simulink library "EngineSystemSubmodelVer1_0"  (R2013a)
settings: Solver=ode45  StartTime=0.0  StopTime=10.0  FixedStep=1e-4  RelTol=1e-3
values from neighbouring files (symbols this model uses):
  B = [B1;B2]    [GensetRespOptimiztion.m]    (also in GensetRespOptimiztionTorstein.m; Init8RTFLEX68D.m = 0.68; init_MVM.m = 0.127)
  beta = 0.75    [Init8RTFLEX68D.m]
  cAStartRef = 104.8    [Init8RTFLEX68D.m]
  coeffMechEff = [0.135;0.155]    [Init8RTFLEX68D.m]
  comp_eff_map = [0 0 0 0 0 0 0 0 0 0 0 0 ... (250000 elements, 500x500)]    [comp_map.mat]    (also in comp_mapABB A175-35L.mat)
  comp_flow_map = [0 0 0 0 0 0 0 0 0 0 0 0 ... (250000 elements, 500x500)]    [comp_map.mat]    (also in comp_mapABB A175-35L.mat)
  D_turb_wheel = TC.TC_map.turb.D_wheel    [init_MVM.m]
  dCALiftDown = cAVVDownRef(end) - cAVVDownRef(1)    [Init8RTFLEX68D.m]
  dCALiftTopRef = 63.5    [Init8RTFLEX68D.m]
  dCALiftUp = cAVVUpRef(end) - cAVVUpRef(1)    [Init8RTFLEX68D.m]
  Dp = 0.383    [Init8RTFLEX68D.m]
  Ds = 0.079    [Init8RTFLEX68D.m]
  Dv = 0.425    [Init8RTFLEX68D.m]
  eff_coeff = [-1.0889528323728;0.91854258409396;-0.10659748546926;                     0.21229452390244;-0.053186221596493;-0.005451194709834]    [Init8RTFLEX68D.m]
  eta_turb_max = TC.TC_map.turb.eff_max    [init_MVM.m]
  flow_coeff_turb = [-1.585326540339;-4.823836967181;1.5853156139822]    [Init8RTFLEX68D.m]    (also in init_MVM.m = TC.TC_map.turb.flow_fit_coeff)
  fs = 0.0683    [Init8RTFLEX68D.m]    (also in NOxProcessGUI.m = varargin{2}; initHybrid.m; initMV.m; init_MVM.m = 0.0682925799315)
  genset = generators(1)    [runTempCyl4S.m]
  J_tc = TC.SAE_map_comp.inertia    [init_MVM.m]
  jShaft = 0    [EngineSystemParameters.m]    (also in Init8RTFLEX68D.m = 323000)
  jTC = 2    [Init8RTFLEX68D.m]
  Kb = 1*ones(engines,1)    [initHybrid.m]    (also in initMV.m; init_MVM.m = 1; init_ele.m = 1)
  Kd = 20*ones(engines,1)    [initHybrid.m]    (also in initMV.m; init_MVM.m = 10; init_ele.m = 20)
  Ki = 20*ones(engines,1)    [initHybrid.m]    (also in initMV.m; init_MVM.m = 10; init_ele.m = 20)
  Kp = 20*ones(engines,1)    [initHybrid.m]    (also in initMV.m; init_MVM.m = 10; init_ele.m = 20)
  lambdaCrank = 0.5056    [Init8RTFLEX68D.m]
  liftMax = 0.17    [Init8RTFLEX68D.m]
  Load_amp = x(4) + xRef(i)    [GetErrGensetResp.m]    (also in runsimulation.m = 0.55; runsimulationRecovery.m = InitialLoad(jj) + LoadStep(ii))
  Load_bias = x(4)    [GetErrGensetResp.m]    (also in runsimulation.m = 0.15; runsimulationRecovery.m = InitialLoad(jj))
  Load_index = 1    [GetErrGensetResp.m]    (also in runsimulation.m; runsimulationRecovery.m)
  mqfCycMax = 9.5547e-2    (= 0.095547)    [Init8RTFLEX68D.m]
  N = x*noMol    [NOxProcessGUI.m]    (also in initHybrid.m = .1*ones(engines,1); initMV.m = .1*ones(engines,1); init_ele.m = 0.1)
  n288_rep = [0 222.054 444.108 666.162 888.216 1110.27 1332.324 1554.378 1776.432 1998.486 2220.54 2442.594 ... (500 elements, 1x500)]    [comp_map.mat]
  nPort = 28    [Init8RTFLEX68D.m]
  npr = length(pr_rep)    [Init8RTFLEX68D.m]    (also in initHybrid.m; initMV.m; init_MVM.m)
  nsp = length(n288_rep)    [Init8RTFLEX68D.m]    (also in initHybrid.m; initMV.m; init_MVM.m)
  nStroke = 2    [Init8RTFLEX68D.m]
  omegat0 = RPM_TC_initial/30*pi    [init_MVM.m]
  pr_rep = [1.01 1.0150249672 1.0200499344 1.0250749016 1.0300998688 1.035124836 1.0401498032 1.0451747704 1.0501997376 1.0552247048 1.060249672 1.0652746392 ... (500 elements, 1x500)]    [comp_map.mat]
  r = 0.035    [Init8RTFLEX68D.m]
  Start_time = 50    [GetErrGensetResp.m]    (also in runsimulation.m; runsimulationRecovery.m)
  stroke = 2.72    [Init8RTFLEX68D.m]
  T_load = 1    [GetErrGensetResp.m]    (also in runsimulation.m; runsimulationRecovery.m)
  T_ref_turb = TC.TC_map.turb.T_ref    [init_MVM.m]
  u0 = 0.2    [init_MVM.m]
  Uc_opt = TC.TC_map.turb.Uc_opt    [init_MVM.m]
  w = 0.021    [Init8RTFLEX68D.m]
  wasteGateMax = 10    [Init8RTFLEX68D.m]
  wasteGateMin = 0    [Init8RTFLEX68D.m]
  wiebePara = [0.07;0.57;3.05;11;24;56.3;1.5;1;0.7]    [Init8RTFLEX68D.m]
  X = 0.07    [Init8RTFLEX68D.m]
  Y = 0.16    [Init8RTFLEX68D.m]
undefined symbols (not defined in the file or in its folder): aCrank, cAVVDownRef, cAVVUpRef, liftDownRef, liftUpRef, omega0, Td, Ti, u_max
undefined symbols (not defined in the file): BWdmExhBypass, cAlpha, cCylHT, E0A, ECyl0, hn, KbWG, KpWG, lowerCloseSPWG, m0A, mb0A, mbCyl0, mCp, mCyl0, nCyl, phi0, phi0A, phi0rad, RPM0, RPMMax, RPMT0, TiWG, upperOpenWG, V0A, vCyl0, wasteGateRatio
libraries: EngineSystemSubmodel x49, simulink x1
(part 2 of 3)

== system EngineSystemSubmodelVer1_0/AirWaterCooler ==
  pTFu : Inport
  pTFd : Inport  Port=2
  TCW : Inport  Port=3
  Demux : Demux  Outputs=3
  Demux1 : Demux  Outputs=3
  Mux : Mux  Inputs=3
  Mux1 : Mux  Inputs=3
  S-Function : S-Function  FunctionName=AirWaterCoolerPTF  Parameters=fs,Cd,A_air_path,dm_cw,coeff_T_cw_K,Cp_cw,D_cw_pipe  SFunctionModules='GetAirDensity GetAirThermalConduct GetAirViscosity GetCompCombGas_rtwutil GetHTCoeffHTX GetIdealNozzleFlow GetThdynCombGasZach rt_nonfinite rtGetInf rtGetNaN'  EnableBusSupport=off  mask{fs=fs, Cd=Cd, A_air_path=A_air_path, dm_cw=dm_cw, coeff_T_cw_K=coeff_T_cw_K, Cp_cw=Cp_cw, D_cw_pipe=D_cw_pipe}
      mask prompts: fs "Stoichiometric fuel-air ratio"; Cd "Discharge coefficient (0.8)"; A_air_path "Effective sectional area of air path (m2)"; dm_cw "Coolant flow rate (kg/s)"; coeff_T_cw_K "Coefficient for effective heat transfer area w.r.t. coolant temperature (2x1)"; Cp_cw "Specific heat capacity of coolant"; D_cw_pipe "Pipe diameter of the cooling water pipe in the cooler (m)"
  dmEmbu : Outport
  dmEmbd : Outport  Port=2
  wires:
  S-Function/6 -> Mux1/3
  S-Function/5 -> Mux1/2
  S-Function/4 -> Mux1/1
  S-Function/3 -> Mux/3
  S-Function/2 -> Mux/2
  S-Function/1 -> Mux/1
  Demux/1 -> S-Function/1
  Demux/3 -> S-Function/3
  Demux/2 -> S-Function/2
  Demux1/3 -> S-Function/6
  Demux1/1 -> S-Function/4
  Demux1/2 -> S-Function/5
  pTFd/1 -> Demux1/1
  pTFu/1 -> Demux/1
  Mux/1 -> dmEmbu/1
  Mux1/1 -> dmEmbd/1
  TCW/1 -> S-Function/7

== system EngineSystemSubmodelVer1_0/AirWaterCoolerNV ==
  pTFu : Inport
  pTFd : Inport  Port=2
  TCW : Inport  Port=3
  Bus Creator : BusCreator  Inputs=3
  Bus Creator1 : BusCreator  Inputs=3
  Bus Selector : BusSelector  OutputSignals=p,T,F
  Bus Selector1 : BusSelector  OutputSignals=p,T,F
  S-Function : S-Function  FunctionName=AirWaterCoolerPTF  Parameters=fs,Cd,A_air_path,dm_cw,coeff_T_cw_K,Cp_cw,D_cw_pipe  SFunctionModules='GetAirDensity GetAirThermalConduct GetAirViscosity GetCompCombGas_rtwutil GetHTCoeffHTX GetIdealNozzleFlow GetThdynCombGasZach rt_nonfinite rtGetInf rtGetNaN'  EnableBusSupport=off  mask{fs=fs, Cd=Cd, A_air_path=A_air_path, dm_cw=dm_cw, coeff_T_cw_K=coeff_T_cw_K, Cp_cw=Cp_cw, D_cw_pipe=D_cw_pipe}
      mask prompts: fs "Stoichiometric fuel-air ratio"; Cd "Discharge coefficient (0.8)"; A_air_path "Effective sectional area of air path (m2)"; dm_cw "Coolant flow rate (kg/s)"; coeff_T_cw_K "Coefficient for effective heat transfer area w.r.t. coolant temperature (2x1)"; Cp_cw "Specific heat capacity of coolant"; D_cw_pipe "Pipe diameter of the cooling water pipe in the cooler (m)"
  dmEmbu : Outport
  dmEmbd : Outport  Port=2
  wires:
  TCW/1 -> S-Function/7
  S-Function/1 -> Bus Creator/1  "dmu"
  S-Function/2 -> Bus Creator/2  "dEu"
  S-Function/3 -> Bus Creator/3  "dmbu"
  Bus Creator/1 -> dmEmbu/1
  S-Function/5 -> Bus Creator1/2  "dEd"
  S-Function/6 -> Bus Creator1/3  "dmbd"
  S-Function/4 -> Bus Creator1/1  "dmd"
  Bus Creator1/1 -> dmEmbd/1
  pTFu/1 -> Bus Selector/1
  pTFd/1 -> Bus Selector1/1
  Bus Selector/1 -> S-Function/1  "<p>"
  Bus Selector/2 -> S-Function/2  "<T>"
  Bus Selector/3 -> S-Function/3  "<F>"
  Bus Selector1/2 -> S-Function/5  "<T>"
  Bus Selector1/1 -> S-Function/4  "<p>"
  Bus Selector1/3 -> S-Function/6  "<F>"

== system EngineSystemSubmodelVer1_0/Compressor ==
  pTF_u : Inport
  pTF_d : Inport  Port=2
  omegat : Inport  Port=3
  Demux : Demux  Outputs=3
  Demux1 : Demux  Outputs=3
  Mux : Mux  Inputs=3
  Mux1 : Mux  Inputs=3
  S-Function : S-Function  FunctionName=compressor_calc_PTF  Parameters=fs,comp_flow_map,comp_eff_map,pr_rep,n288_rep,int32(npr),int32(nsp)  SFunctionModules=GetThdynCombGasZach.c  EnableBusSupport=off
  dmEmb_u : Outport
  dmEmb_d : Outport  Port=2
  Tqt : Outport  Port=3
  eta_c : Outport  Port=4
  wires:
  Demux/1 -> S-Function/1
  Demux/3 -> S-Function/3
  Demux/2 -> S-Function/2
  Demux1/2 -> S-Function/5
  Demux1/3 -> S-Function/6
  Demux1/1 -> S-Function/4
  pTF_d/1 -> Demux1/1
  omegat/1 -> S-Function/7
  pTF_u/1 -> Demux/1
  S-Function/5 -> Mux1/2
  S-Function/4 -> Mux1/1
  S-Function/6 -> Mux1/3
  S-Function/1 -> Mux/1
  S-Function/2 -> Mux/2
  S-Function/3 -> Mux/3
  Mux/1 -> dmEmb_u/1
  Mux1/1 -> dmEmb_d/1
  S-Function/7 -> Tqt/1
  S-Function/8 -> eta_c/1

== system EngineSystemSubmodelVer1_0/CompressorNV ==
  pTF_u : Inport
  pTF_d : Inport  Port=2
  omegat : Inport  Port=3
  Bus Creator : BusCreator  Inputs=3
  Bus Creator1 : BusCreator  Inputs=3
  Bus Selector : BusSelector  OutputSignals=p,T,F
  Bus Selector1 : BusSelector  OutputSignals=p,T,F
  S-Function : S-Function  FunctionName=compressor_calc_PTF  Parameters=fs,comp_flow_map,comp_eff_map,pr_rep,n288_rep,int32(npr),int32(nsp)  SFunctionModules=GetThdynCombGasZach.c  EnableBusSupport=off
  dmEmb_u : Outport
  dmEmb_d : Outport  Port=2
  Tqt : Outport  Port=3
  eta_c : Outport  Port=4
  wires:
  pTF_d/1 -> Bus Selector1/1
  pTF_u/1 -> Bus Selector/1
  Bus Selector/2 -> S-Function/2  "<T>"
  Bus Selector/3 -> S-Function/3  "<F>"
  Bus Selector/1 -> S-Function/1  "<p>"
  Bus Selector1/2 -> S-Function/5  "<T>"
  Bus Selector1/3 -> S-Function/6  "<F>"
  Bus Selector1/1 -> S-Function/4  "<p>"
  omegat/1 -> S-Function/7
  S-Function/2 -> Bus Creator/2  "dEu"
  S-Function/1 -> Bus Creator/1  "dmu"
  S-Function/3 -> Bus Creator/3  "dmbu"
  S-Function/5 -> Bus Creator1/2  "dEd"
  S-Function/4 -> Bus Creator1/1  "dmd"
  S-Function/6 -> Bus Creator1/3  "dmbd"
  S-Function/7 -> Tqt/1
  S-Function/8 -> eta_c/1
  Bus Creator/1 -> dmEmb_u/1
  Bus Creator1/1 -> dmEmb_d/1

== system EngineSystemSubmodelVer1_0/CrankMechKinematic ==
  pCyl : Inport
  omega : Inport  Port=2
  pScav : Inport  Port=3
  S-Function : S-Function  FunctionName=crankMechKinematic  Parameters=phi0, B, stroke, lambdaCrank  EnableBusSupport=off  mask{phi0=phi0, B=B, stroke=stroke, lambdaCrank=lambdaCrank}
      mask prompts: phi0 "Initial crank angle"; B "Bore of the cylinder"; lambdaCrank "Ratio of length of crank rod to that of connecting rod"
  pow : Outport
  dV : Outport  Port=2
  Tq : Outport  Port=3
  phi : Outport  Port=4
  wires:
  omega/1 -> S-Function/2
  pScav/1 -> S-Function/3
  pCyl/1 -> S-Function/1
  S-Function/4 -> phi/1
  S-Function/3 -> pow/1
  S-Function/2 -> Tq/1
  S-Function/1 -> dV/1

== system EngineSystemSubmodelVer1_0/EngCylHeatTransfer ==
  omega : Inport
  pTFV_Cyl : Inport  Port=2
  Bus Selector : BusSelector  OutputSignals=p,T,V
  S-Function : S-Function  FunctionName=EngCylHeatTransfer  Parameters=stroke, B, cAlpha, mCp, tempWall0, cCylHT, nCyl  EnableBusSupport=off  mask{stroke=stroke, B=B, cAlpha=cAlpha, mCp=mCp, cCylHT=cCylHT, nCyl=nCyl, tempWall0=tempWall0}
      mask prompts: stroke "Storke [m]"; B "Bore [m]"; cAlpha "Fitting coefficient for convective heat transfer coefficient"; mCp "Heat capacity of the cylinder [J/K]"; cCylHT "Polynomial coefficient for heat rejection model from the cylinder (4 x 1)"; nCyl "Number of cylinders"; tempWall0 "Initial cylinder wall temperature"
  dQ : Outport
  tempWall : Outport  Port=2
  wires:
  Bus Selector/3 -> S-Function/3  "<V>"
  Bus Selector/1 -> S-Function/1  "<p>"
  Bus Selector/2 -> S-Function/2  "<T>"
  omega/1 -> S-Function/4
  pTFV_Cyl/1 -> Bus Selector/1
  S-Function/2 -> tempWall/1
  S-Function/1 -> dQ/1

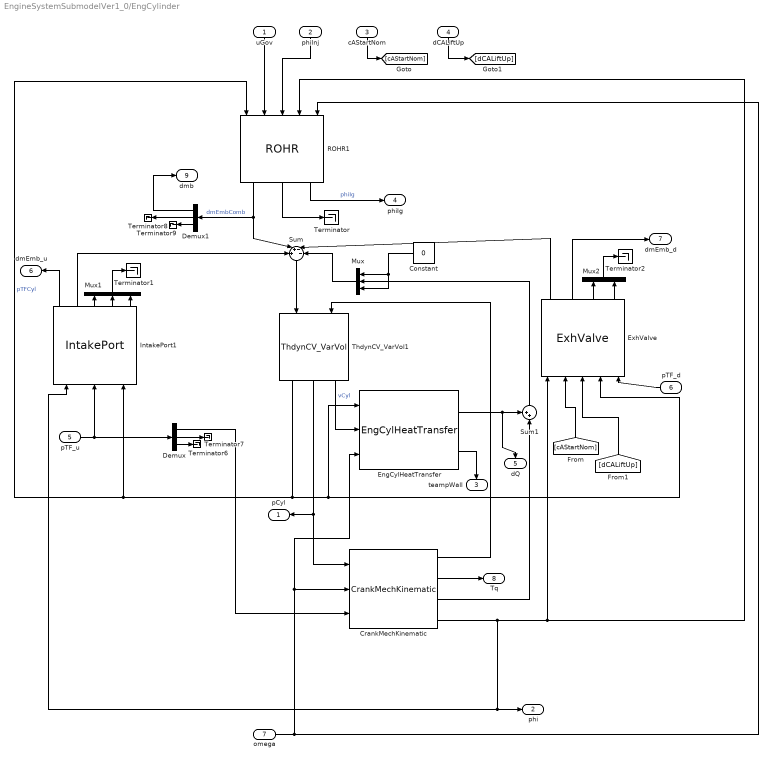
== system EngineSystemSubmodelVer1_0/EngCylinder ==
  uGov : Inport
  phiInj : Inport  Port=2
  cAStartNom : Inport  Port=3
  dCALiftUp : Inport  Port=4
  pTF_u : Inport  Port=5
  pTF_d : Inport  Port=6
  omega : Inport  Port=7
  Constant : Constant  Value=0
  CrankMechKinematic : EngineSystemSubmodel/CrankMechKinematic  phi0=phi0  B=B  stroke=stroke  lambdaCrank=lambdaCrank
  Demux : Demux  Outputs=3
  Demux1 : Demux  Outputs=3
  EngCylHeatTransfer : EngineSystemSubmodel/EngCylHeatTransfer  stroke=stroke  B=B  cAlpha=cAlpha  mCp=mCp  cCylHT=cCylHT  nCyl=nCyl  tempWall0=600
  ExhValve : EngineSystemSubmodel/ExhValve  fs=fs  cAVVUpRef=cAVVUpRef  cAVVDownRef=cAVVDownRef  liftUpRef=liftUpRef  liftDownRef=liftDownRef  cAStartRef=cAStartRef  dCALiftUp=dCALiftUp  dCALiftDown=dCALiftDown  dCALiftTopRef=dCALiftTopRef  liftMax=liftMax  Dv=Dv  beta=beta  w=w  Dp=Dp  Ds=Ds
  IntakePort1 : EngineSystemSubmodel/IntakePort  fs=fs  nStroke=nStroke  aCrank=aCrank  lambdaCrank=lambdaCrank  X=X  Y=Y  r=r  nPort=nPort  stroke=stroke
  Mux : Mux  Inputs=3
  Mux1 : Mux  Inputs=3
  Mux2 : Mux  Inputs=2
  ROHR1 : EngineSystemSubmodel/ROHR  mqfCycMax=mqfCycMax  wiebePara=wiebePara  hn=hn
  Sum : Sum  Inputs=++--
  Sum1 : Sum  Inputs=++|
  Terminator{,1..2,6..9} (7 alike) : Terminator
  ThdynCV_VarVol1 : EngineSystemSubmodel/ThdynCV_VarVol  fs=fs  m0=m0  E0=E0  mb0=mb0  V0=V0
  pCyl : Outport
  phi : Outport  Port=2
  teampWall : Outport  Port=3
  phiIg : Outport  Port=4
  dQ : Outport  Port=5
  dmEmb_u : Outport  Port=6
  dmEmb_d : Outport  Port=7
  Tq : Outport  Port=8
  dmb : Outport  Port=9
  wires:
  [dCALiftUp] -> ExhValve/3
  [cAStartNom] -> ExhValve/2
  dCALiftUp/1 -> [dCALiftUp]
  cAStartNom/1 -> [cAStartNom]
  ExhValve/2 -> dmEmb_d/1
  Mux2/1 -> Terminator2/1
  ExhValve/4 -> Mux2/2
  ExhValve/3 -> Mux2/1
  Mux1/1 -> Terminator1/1
  IntakePort1/5 -> Mux1/3
  IntakePort1/4 -> Mux1/2
  IntakePort1/3 -> Mux1/1
  ROHR1/3 -> phiIg/1  "phiIg"
  EngCylHeatTransfer/2 -> teampWall/1
  Demux/3 -> Terminator7/1
  Demux/2 -> Terminator6/1
  Constant/1 -> Mux/1, Mux/3
  Mux/1 -> Sum/4
  Sum1/1 -> Mux/2
  EngCylHeatTransfer/1 -> dQ/1, Sum1/1
  ThdynCV_VarVol1/3 -> EngCylHeatTransfer/2  "vCyl"
  pTF_u/1 -> Demux/1, IntakePort1/2
  IntakePort1/1 -> dmEmb_u/1
  ROHR1/2 -> Terminator/1
  omega/1 -> ROHR1/5, CrankMechKinematic/2, EngCylHeatTransfer/3
  pTF_d/1 -> ExhValve/5
  phiInj/1 -> ROHR1/3
  CrankMechKinematic/2 -> Tq/1
  Demux/1 -> CrankMechKinematic/3
  CrankMechKinematic/3 -> Sum1/2
  uGov/1 -> ROHR1/2
  CrankMechKinematic/1 -> ThdynCV_VarVol1/2
  CrankMechKinematic/4 -> IntakePort1/1, phi/1, ExhValve/1, ROHR1/4
  ThdynCV_VarVol1/2 -> CrankMechKinematic/1, pCyl/1
  ThdynCV_VarVol1/1 -> IntakePort1/3, ROHR1/1, ExhValve/4, EngCylHeatTransfer/1  "pTFCyl"
  Sum/1 -> ThdynCV_VarVol1/1
  ExhValve/1 -> Sum/3
  IntakePort1/2 -> Sum/1
  ROHR1/1 -> Sum/2, Demux1/1  "dmEmbComb"
  Demux1/1 -> dmb/1
  Demux1/2 -> Terminator8/1
  Demux1/3 -> Terminator9/1

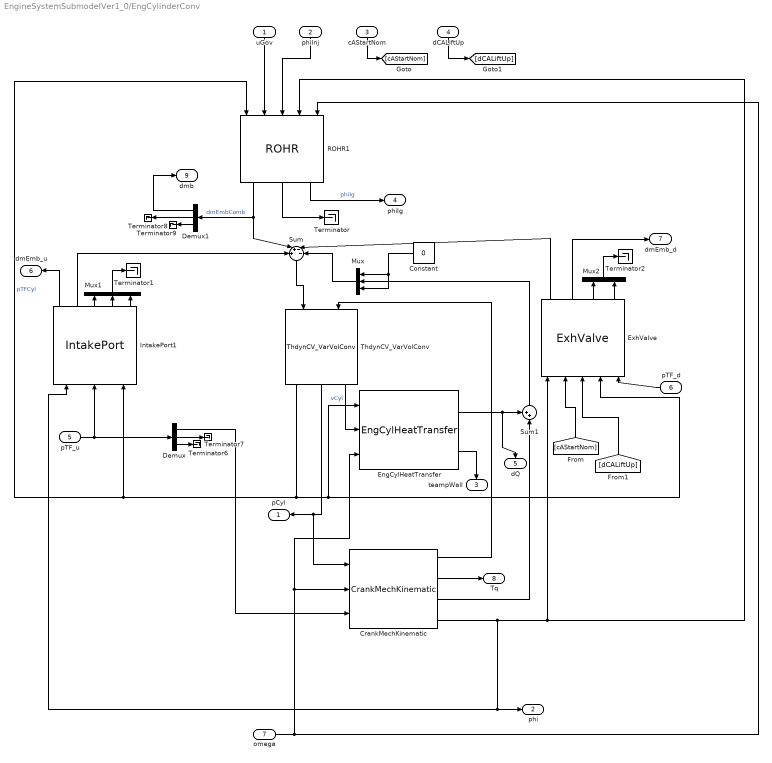
== system EngineSystemSubmodelVer1_0/EngCylinderConv ==
  uGov : Inport
  phiInj : Inport  Port=2
  cAStartNom : Inport  Port=3
  dCALiftUp : Inport  Port=4
  pTF_u : Inport  Port=5
  pTF_d : Inport  Port=6
  omega : Inport  Port=7
  Constant : Constant  Value=0
  CrankMechKinematic : EngineSystemSubmodel/CrankMechKinematic  phi0=phi0  B=B  stroke=stroke  lambdaCrank=lambdaCrank
  Demux : Demux  Outputs=3
  Demux1 : Demux  Outputs=3
  EngCylHeatTransfer : EngineSystemSubmodel/EngCylHeatTransfer  stroke=stroke  B=B  cAlpha=cAlpha  mCp=mCp  cCylHT=cCylHT  nCyl=nCyl  tempWall0=600
  ExhValve : EngineSystemSubmodel/ExhValve  fs=fs  cAVVUpRef=cAVVUpRef  cAVVDownRef=cAVVDownRef  liftUpRef=liftUpRef  liftDownRef=liftDownRef  cAStartRef=cAStartRef  dCALiftUp=dCALiftUp  dCALiftDown=dCALiftDown  dCALiftTopRef=dCALiftTopRef  liftMax=liftMax  Dv=Dv  beta=beta  w=w  Dp=Dp  Ds=Ds
  IntakePort1 : EngineSystemSubmodel/IntakePort  fs=fs  nStroke=nStroke  aCrank=aCrank  lambdaCrank=lambdaCrank  X=X  Y=Y  r=r  nPort=nPort  stroke=stroke
  Mux : Mux  Inputs=3
  Mux1 : Mux  Inputs=3
  Mux2 : Mux  Inputs=2
  ROHR1 : EngineSystemSubmodel/ROHR  mqfCycMax=mqfCycMax  wiebePara=wiebePara  hn=hn
  Sum : Sum  Inputs=++--
  Sum1 : Sum  Inputs=++|
  Terminator{,1..2,6..9} (7 alike) : Terminator
  ThdynCV_VarVolConv : EngineSystemSubmodel/ThdynCV_VarVolConv  fs=fs  p0=p0  T0=T0  F0=F0  V0=V0
  pCyl : Outport
  phi : Outport  Port=2
  teampWall : Outport  Port=3
  phiIg : Outport  Port=4
  dQ : Outport  Port=5
  dmEmb_u : Outport  Port=6
  dmEmb_d : Outport  Port=7
  Tq : Outport  Port=8
  dmb : Outport  Port=9
  wires:
  [dCALiftUp] -> ExhValve/3
  [cAStartNom] -> ExhValve/2
  dCALiftUp/1 -> [dCALiftUp]
  cAStartNom/1 -> [cAStartNom]
  ExhValve/2 -> dmEmb_d/1
  Mux2/1 -> Terminator2/1
  ExhValve/4 -> Mux2/2
  ExhValve/3 -> Mux2/1
  Mux1/1 -> Terminator1/1
  IntakePort1/5 -> Mux1/3
  IntakePort1/4 -> Mux1/2
  IntakePort1/3 -> Mux1/1
  ROHR1/3 -> phiIg/1  "phiIg"
  EngCylHeatTransfer/2 -> teampWall/1
  Demux/3 -> Terminator7/1
  Demux/2 -> Terminator6/1
  Constant/1 -> Mux/1, Mux/3
  Mux/1 -> Sum/4
  Sum1/1 -> Mux/2
  EngCylHeatTransfer/1 -> dQ/1, Sum1/1
  ThdynCV_VarVolConv/3 -> EngCylHeatTransfer/2  "vCyl"
  pTF_u/1 -> Demux/1, IntakePort1/2
  IntakePort1/1 -> dmEmb_u/1
  ROHR1/2 -> Terminator/1
  omega/1 -> ROHR1/5, CrankMechKinematic/2, EngCylHeatTransfer/3
  pTF_d/1 -> ExhValve/5
  phiInj/1 -> ROHR1/3
  CrankMechKinematic/2 -> Tq/1
  Demux/1 -> CrankMechKinematic/3
  CrankMechKinematic/3 -> Sum1/2
  uGov/1 -> ROHR1/2
  CrankMechKinematic/1 -> ThdynCV_VarVolConv/2
  CrankMechKinematic/4 -> IntakePort1/1, phi/1, ExhValve/1, ROHR1/4
  ThdynCV_VarVolConv/2 -> pCyl/1, CrankMechKinematic/1
  ThdynCV_VarVolConv/1 -> IntakePort1/3, ROHR1/1, ExhValve/4, EngCylHeatTransfer/1  "pTFCyl"
  Sum/1 -> ThdynCV_VarVolConv/1
  ExhValve/1 -> Sum/3
  IntakePort1/2 -> Sum/1
  ROHR1/1 -> Sum/2, Demux1/1  "dmEmbComb"
  Demux1/1 -> dmb/1
  Demux1/2 -> Terminator8/1
  Demux1/3 -> Terminator9/1

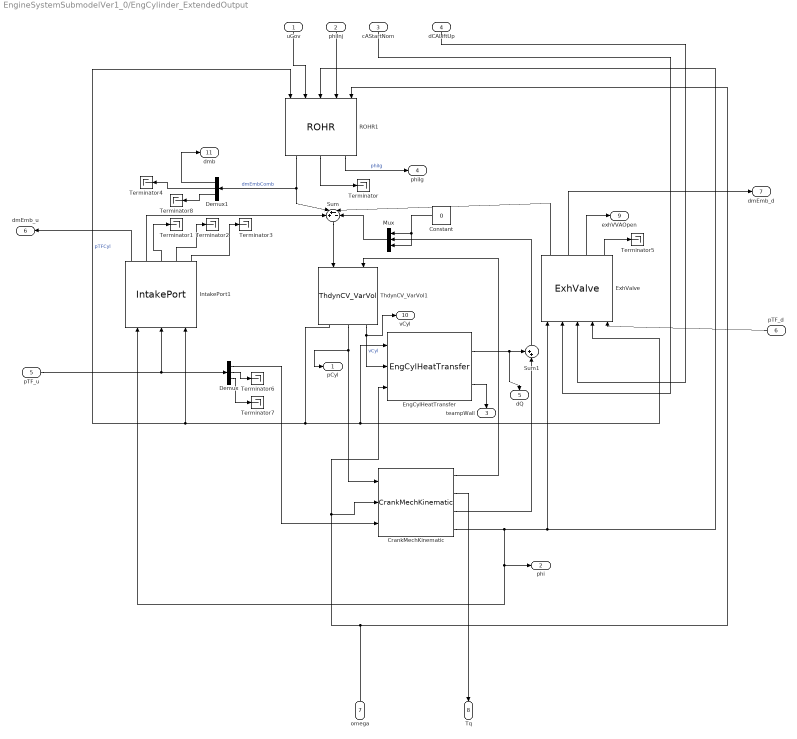
== system EngineSystemSubmodelVer1_0/EngCylinder_ExtendedOutput ==
  uGov : Inport
  phiInj : Inport  Port=2
  cAStartNom : Inport  Port=3
  dCALiftUp : Inport  Port=4
  pTF_u : Inport  Port=5
  pTF_d : Inport  Port=6
  omega : Inport  Port=7
  Constant : Constant  Value=0
  CrankMechKinematic : EngineSystemSubmodel/CrankMechKinematic  phi0=phi0  B=B  stroke=stroke  lambdaCrank=lambdaCrank
  Demux : Demux  Outputs=3
  Demux1 : Demux  Outputs=3
  EngCylHeatTransfer : EngineSystemSubmodel/EngCylHeatTransfer  stroke=stroke  B=B  cAlpha=cAlpha  mCp=mCp  cCylHT=cCylHT  nCyl=nCyl  tempWall0=350
  ExhValve : EngineSystemSubmodel/ExhValve  fs=fs  cAVVUpRef=cAVVUpRef  cAVVDownRef=cAVVDownRef  liftUpRef=liftUpRef  liftDownRef=liftDownRef  cAStartRef=cAStartRef  dCALiftUp=dCALiftUp  dCALiftDown=dCALiftDown  dCALiftTopRef=dCALiftTopRef  liftMax=liftMax  Dv=Dv  beta=beta  w=w  Dp=Dp  Ds=Ds
  IntakePort1 : EngineSystemSubmodel/IntakePort  fs=fs  nStroke=nStroke  aCrank=aCrank  lambdaCrank=lambdaCrank  X=X  Y=Y  r=r  nPort=nPort  stroke=stroke
  Mux : Mux  Inputs=3
  ROHR1 : EngineSystemSubmodel/ROHR  mqfCycMax=mqfCycMax  wiebePara=wiebePara  hn=hn
  Sum : Sum  Inputs=++--
  Sum1 : Sum  Inputs=++|
  Terminator{,1..8} (9 alike) : Terminator
  ThdynCV_VarVol1 : EngineSystemSubmodel/ThdynCV_VarVol  fs=fs  m0=m0  E0=E0  mb0=mb0  V0=V0
  pCyl : Outport
  phi : Outport  Port=2
  teampWall : Outport  Port=3
  phiIg : Outport  Port=4
  dQ : Outport  Port=5
  dmEmb_u : Outport  Port=6
  dmEmb_d : Outport  Port=7
  Tq : Outport  Port=8
  exhVVAOpen : Outport  Port=9
  vCyl : Outport  Port=10
  dmb : Outport  Port=11
  wires:
  IntakePort1/2 -> Sum/1
  ExhValve/1 -> Sum/3
  ROHR1/1 -> Demux1/1, Sum/2  "dmEmbComb"
  Sum/1 -> ThdynCV_VarVol1/1
  ThdynCV_VarVol1/1 -> EngCylHeatTransfer/1, ExhValve/4, ROHR1/1, IntakePort1/3  "pTFCyl"
  ThdynCV_VarVol1/2 -> CrankMechKinematic/1, pCyl/1
  CrankMechKinematic/4 -> ROHR1/3, ExhValve/1, phi/1, IntakePort1/1
  CrankMechKinematic/1 -> ThdynCV_VarVol1/2
  cAStartNom/1 -> ExhValve/2
  uGov/1 -> ROHR1/2
  CrankMechKinematic/3 -> Sum1/2
  ExhValve/4 -> Terminator5/1
  Demux/1 -> CrankMechKinematic/3
  CrankMechKinematic/2 -> Tq/1
  phiInj/1 -> ROHR1/4
  pTF_d/1 -> ExhValve/5
  omega/1 -> ROHR1/5, EngCylHeatTransfer/3, CrankMechKinematic/2
  ROHR1/2 -> Terminator/1
  IntakePort1/1 -> dmEmb_u/1
  IntakePort1/3 -> Terminator1/1
  dCALiftUp/1 -> ExhValve/3
  IntakePort1/5 -> Terminator3/1
  ExhValve/3 -> exhVVAOpen/1
  pTF_u/1 -> IntakePort1/2, Demux/1
  IntakePort1/4 -> Terminator2/1
  ExhValve/2 -> dmEmb_d/1
  ThdynCV_VarVol1/3 -> vCyl/1, EngCylHeatTransfer/2  "vCyl"
  EngCylHeatTransfer/1 -> Sum1/1, dQ/1
  Sum1/1 -> Mux/2
  Mux/1 -> Sum/4
  Constant/1 -> Mux/3, Mux/1
  Demux/2 -> Terminator6/1
  Demux/3 -> Terminator7/1
  EngCylHeatTransfer/2 -> teampWall/1
  ROHR1/3 -> phiIg/1  "phiIg"
  Demux1/1 -> dmb/1
  Demux1/2 -> Terminator4/1
  Demux1/3 -> Terminator8/1

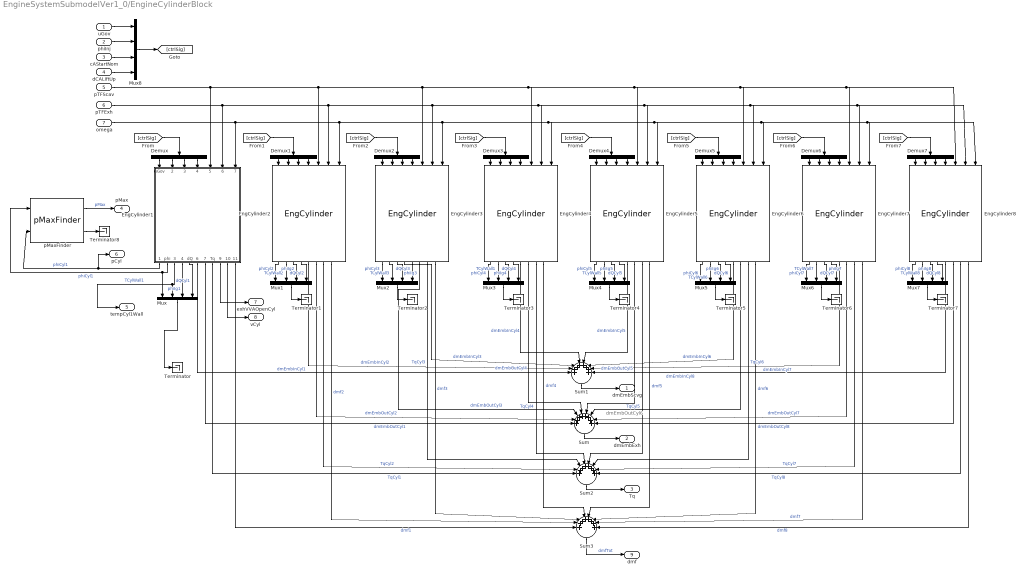
== system EngineSystemSubmodelVer1_0/EngineCylinderBlock ==
  note: dmEmbOutCyl6
  uGov : Inport
  phiInj : Inport  Port=2
  cAStartNom : Inport  Port=3
  dCALiftUp : Inport  Port=4
  pTFScav : Inport  Port=5
  pTFExh : Inport  Port=6
  omega : Inport  Port=7
  Demux{,1..7} (8 alike) : Demux
  EngCylinder1 : Subsystem  AncestorBlock=EngineSystemSubmodel/EngCylinder_ExtendedOutput  mask{fs=fs, nStroke=nStroke, hn=hn, nCyl=nCyl, iCyl=1, B=B, stroke=stroke, lambdaCrank=lambdaCrank, aCrank=aCrank, X=X, Y=Y, r=r, nPort=nPort, liftMax=liftMax, Dv=Dv, beta=beta, w=w, Dp=Dp, Ds=Ds, cAVVUpRef=cAVVUpRef, cAVVDownRef=cAVVDownRef, liftUpRef=liftUpRef, liftDownRef=liftDownRef, cAStartRef=cAStartRef, dCALiftUp=dCALiftUp, dCALiftDown=dCALiftDown, dCALiftTopRef=dCALiftTopRef, mCp=mCp, cCylHT=cCylHT, cAlpha=cAlpha, mqfCycMax=mqfCycMax, wiebePara=wiebePara, phi0=phi0, m0=mCyl0, E0=ECyl0, mb0=mbCyl0, V0=vCyl0, phi0A=phi0A, m0A=m0A, E0A=E0A, mb0A=mb0A, V0A=V0A}
      mask prompts: fs "Stoichiometric fuel-air ratio"; nStroke "Number of stroke"; hn "Lower heating value of the fuel [J/kg]"; nCyl "Number of cylinders"; iCyl "Cylinder number"; B "Bore of the cylinder [m]"; stroke "Stroke [m]"; lambdaCrank "Ratio of length of crank rod to connecting rod"; aCrank "Length of crank rod [m]"; X "Width of inport opening [m]"; Y "Height of inport opening [m]"; r "Raidus of fillet of the opening"; nPort "Number of ports [pcs]"; liftMax "Maximum valve lift [m]"; Dv "Valve head diameter [m]"; beta "Seat angle [rad]"; w "Valve seat width [m]"; Dp "Inner seat diameter [m]"; Ds "Stem diameter [m]"; cAVVUpRef "Crank angle array for opening [deg]"; cAVVDownRef "Crank angle array for closing [deg]"; liftUpRef "Normalized lift array for opening (0~1)"; liftDownRef "Normalized lift array for closing (0~1)"; cAStartRef "Nominal crank angle at start of valve lif [deg]"; dCALiftUp "Nominal duration of crank angle for valve opening [deg]"; dCALiftDown "Nominal duration of crank angle for valve closing [deg]"; dCALiftTopRef "Nominal duration of crank angle for valve open [deg]"; mCp "Heat capacity of the cylinder [J/K]"; cCylHT "Polynomial coefficient for heat rejection model from the cylinder (4 x 1)"; cAlpha "Fitting coefficient for convective heat transfer coefficient"; mqfCycMax "Maximum fuel mass injected per cycle [kg]"; wiebePara "3-Wiebe Parameters (9x1)"; phi0 "Initial crank angle [deg]"; m0 "Initial mass [kg]"; E0 "Initial internal energy [J]"; mb0 "Initial burned fuel mass [kg]"; V0 "Initial volume [m3]"; phi0A "Initial crank angle array [deg]"; m0A "Initial mass array [kg]"; E0A "Initial internal energy array [J]"; mb0A "Initial burned fuel mass array [kg]"; V0A "Initial volume array [m3]"
      mask init: same as EngineSystemSubmodelVer1_0/EngCylinder
      mask TypeOptions fs: ThdynCV_VarVol1/fs | IntakePort1/fs | ExhValve/fs
      mask TypeOptions nStroke: IntakePort1/nStroke
      mask TypeOptions hn: ROHR1/hn
      mask TypeOptions nCyl: EngCylHeatTransfer/nCyl
      mask TypeOptions B: CrankMechKinematic/B | EngCylHeatTransfer/B
      mask TypeOptions stroke: CrankMechKinematic/stroke | EngCylHeatTransfer/stroke | IntakePort1/stroke
      mask TypeOptions lambdaCrank: IntakePort1/lambdaCrank | CrankMechKinematic/lambdaCrank
      mask TypeOptions aCrank: IntakePort1/aCrank
      mask TypeOptions X: IntakePort1/X
      mask TypeOptions Y: IntakePort1/Y
      mask TypeOptions r: IntakePort1/r
      mask TypeOptions nPort: IntakePort1/nPort
      mask TypeOptions liftMax: ExhValve/liftMax
      mask TypeOptions Dv: ExhValve/Dv
      mask TypeOptions beta: ExhValve/beta
      mask TypeOptions w: ExhValve/w
      mask TypeOptions Dp: ExhValve/Dp
      mask TypeOptions Ds: ExhValve/Ds
      mask TypeOptions cAVVUpRef: ExhValve/cAVVUpRef
      mask TypeOptions cAVVDownRef: ExhValve/cAVVDownRef
      mask TypeOptions liftUpRef: ExhValve/liftUpRef
      mask TypeOptions liftDownRef: ExhValve/liftDownRef
      mask TypeOptions cAStartRef: ExhValve/cAStartRef
      mask TypeOptions dCALiftUp: ExhValve/dCALiftUp
      mask TypeOptions dCALiftDown: ExhValve/dCALiftDown
      mask TypeOptions dCALiftTopRef: ExhValve/dCALiftTopRef
      mask TypeOptions mCp: EngCylHeatTransfer/mCp
      mask TypeOptions cCylHT: EngCylHeatTransfer/cCylHT
      mask TypeOptions cAlpha: EngCylHeatTransfer/cAlpha
      mask TypeOptions mqfCycMax: ROHR1/mqfCycMax
      mask TypeOptions wiebePara: ROHR1/wiebePara
      mask TypeOptions phi0: CrankMechKinematic/phi0
      mask TypeOptions m0: ThdynCV_VarVol1/m0
      mask TypeOptions E0: ThdynCV_VarVol1/E0
      mask TypeOptions mb0: ThdynCV_VarVol1/mb0
      mask TypeOptions V0: ThdynCV_VarVol1/V0
  EngCylinder2 : EngineSystemSubmodel/EngCylinder  fs=fs  nStroke=nStroke  hn=hn  nCyl=nCyl  iCyl=2  B=B  stroke=stroke  lambdaCrank=lambdaCrank  aCrank=aCrank  X=X  Y=Y  r=r  nPort=nPort  liftMax=liftMax  Dv=Dv  beta=beta  w=w  Dp=Dp  Ds=Ds  cAVVUpRef=cAVVUpRef  cAVVDownRef=cAVVDownRef  liftUpRef=liftUpRef  liftDownRef=liftDownRef  cAStartRef=cAStartRef  dCALiftUp=dCALiftUp  dCALiftDown=dCALiftDown  dCALiftTopRef=dCALiftTopRef  mCp=mCp  cCylHT=cCylHT  cAlpha=cAlpha  mqfCycMax=mqfCycMax  wiebePara=wiebePara  phi0=phi0  m0=mCyl0  E0=ECyl0  mb0=mbCyl0  V0=vCyl0  phi0A=phi0A  m0A=m0A  E0A=E0A  mb0A=mb0A  V0A=V0A
  EngCylinder3 : EngineSystemSubmodel/EngCylinder  fs=fs  nStroke=nStroke  hn=hn  nCyl=nCyl  iCyl=3  B=B  stroke=stroke  lambdaCrank=lambdaCrank  aCrank=aCrank  X=X  Y=Y  r=r  nPort=nPort  liftMax=liftMax  Dv=Dv  beta=beta  w=w  Dp=Dp  Ds=Ds  cAVVUpRef=cAVVUpRef  cAVVDownRef=cAVVDownRef  liftUpRef=liftUpRef  liftDownRef=liftDownRef  cAStartRef=cAStartRef  dCALiftUp=dCALiftUp  dCALiftDown=dCALiftDown  dCALiftTopRef=dCALiftTopRef  mCp=mCp  cCylHT=cCylHT  cAlpha=cAlpha  mqfCycMax=mqfCycMax  wiebePara=wiebePara  phi0=phi0  m0=mCyl0  E0=ECyl0  mb0=mbCyl0  V0=vCyl0  phi0A=phi0A  m0A=m0A  E0A=E0A  mb0A=mb0A  V0A=V0A
  EngCylinder4 : EngineSystemSubmodel/EngCylinder  fs=fs  nStroke=nStroke  hn=hn  nCyl=nCyl  iCyl=4  B=B  stroke=stroke  lambdaCrank=lambdaCrank  aCrank=aCrank  X=X  Y=Y  r=r  nPort=nPort  liftMax=liftMax  Dv=Dv  beta=beta  w=w  Dp=Dp  Ds=Ds  cAVVUpRef=cAVVUpRef  cAVVDownRef=cAVVDownRef  liftUpRef=liftUpRef  liftDownRef=liftDownRef  cAStartRef=cAStartRef  dCALiftUp=dCALiftUp  dCALiftDown=dCALiftDown  dCALiftTopRef=dCALiftTopRef  mCp=mCp  cCylHT=cCylHT  cAlpha=cAlpha  mqfCycMax=mqfCycMax  wiebePara=wiebePara  phi0=phi0  m0=mCyl0  E0=ECyl0  mb0=mbCyl0  V0=vCyl0  phi0A=phi0A  m0A=m0A  E0A=E0A  mb0A=mb0A  V0A=V0A
  EngCylinder5 : EngineSystemSubmodel/EngCylinder  fs=fs  nStroke=nStroke  hn=hn  nCyl=nCyl  iCyl=5  B=B  stroke=stroke  lambdaCrank=lambdaCrank  aCrank=aCrank  X=X  Y=Y  r=r  nPort=nPort  liftMax=liftMax  Dv=Dv  beta=beta  w=w  Dp=Dp  Ds=Ds  cAVVUpRef=cAVVUpRef  cAVVDownRef=cAVVDownRef  liftUpRef=liftUpRef  liftDownRef=liftDownRef  cAStartRef=cAStartRef  dCALiftUp=dCALiftUp  dCALiftDown=dCALiftDown  dCALiftTopRef=dCALiftTopRef  mCp=mCp  cCylHT=cCylHT  cAlpha=cAlpha  mqfCycMax=mqfCycMax  wiebePara=wiebePara  phi0=phi0  m0=mCyl0  E0=ECyl0  mb0=mbCyl0  V0=vCyl0  phi0A=phi0A  m0A=m0A  E0A=E0A  mb0A=mb0A  V0A=V0A
  EngCylinder6 : EngineSystemSubmodel/EngCylinder  fs=fs  nStroke=nStroke  hn=hn  nCyl=nCyl  iCyl=6  B=B  stroke=stroke  lambdaCrank=lambdaCrank  aCrank=aCrank  X=X  Y=Y  r=r  nPort=nPort  liftMax=liftMax  Dv=Dv  beta=beta  w=w  Dp=Dp  Ds=Ds  cAVVUpRef=cAVVUpRef  cAVVDownRef=cAVVDownRef  liftUpRef=liftUpRef  liftDownRef=liftDownRef  cAStartRef=cAStartRef  dCALiftUp=dCALiftUp  dCALiftDown=dCALiftDown  dCALiftTopRef=dCALiftTopRef  mCp=mCp  cCylHT=cCylHT  cAlpha=cAlpha  mqfCycMax=mqfCycMax  wiebePara=wiebePara  phi0=phi0  m0=mCyl0  E0=ECyl0  mb0=mbCyl0  V0=vCyl0  phi0A=phi0A  m0A=m0A  E0A=E0A  mb0A=mb0A  V0A=V0A
  EngCylinder7 : EngineSystemSubmodel/EngCylinder  fs=fs  nStroke=nStroke  hn=hn  nCyl=nCyl  iCyl=7  B=B  stroke=stroke  lambdaCrank=lambdaCrank  aCrank=aCrank  X=X  Y=Y  r=r  nPort=nPort  liftMax=liftMax  Dv=Dv  beta=beta  w=w  Dp=Dp  Ds=Ds  cAVVUpRef=cAVVUpRef  cAVVDownRef=cAVVDownRef  liftUpRef=liftUpRef  liftDownRef=liftDownRef  cAStartRef=cAStartRef  dCALiftUp=dCALiftUp  dCALiftDown=dCALiftDown  dCALiftTopRef=dCALiftTopRef  mCp=mCp  cCylHT=cCylHT  cAlpha=cAlpha  mqfCycMax=mqfCycMax  wiebePara=wiebePara  phi0=phi0  m0=mCyl0  E0=ECyl0  mb0=mbCyl0  V0=vCyl0  phi0A=phi0A  m0A=m0A  E0A=E0A  mb0A=mb0A  V0A=V0A
  EngCylinder8 : EngineSystemSubmodel/EngCylinder  fs=fs  nStroke=nStroke  hn=hn  nCyl=nCyl  iCyl=8  B=B  stroke=stroke  lambdaCrank=lambdaCrank  aCrank=aCrank  X=X  Y=Y  r=r  nPort=nPort  liftMax=liftMax  Dv=Dv  beta=beta  w=w  Dp=Dp  Ds=Ds  cAVVUpRef=cAVVUpRef  cAVVDownRef=cAVVDownRef  liftUpRef=liftUpRef  liftDownRef=liftDownRef  cAStartRef=cAStartRef  dCALiftUp=dCALiftUp  dCALiftDown=dCALiftDown  dCALiftTopRef=dCALiftTopRef  mCp=mCp  cCylHT=cCylHT  cAlpha=cAlpha  mqfCycMax=mqfCycMax  wiebePara=wiebePara  phi0=phi0  m0=mCyl0  E0=ECyl0  mb0=mbCyl0  V0=vCyl0  phi0A=phi0A  m0A=m0A  E0A=E0A  mb0A=mb0A  V0A=V0A
  Mux{,1..8} (9 alike) : Mux
  Sum{,1..3} (4 alike) : Sum  Inputs=++++++++
  Terminator{,1..8} (9 alike) : Terminator
  pMaxFinder : EngineSystemSubmodel/pMaxFinder
  dmEmbScvg : Outport
  dmEmbExh : Outport  Port=2
  Tq : Outport  Port=3
  pMax : Outport  Port=4
  tempCyl1Wall : Outport  Port=5
  pCyl : Outport  Port=6
  exhVVAOpenCyl : Outport  Port=7
  vCyl : Outport  Port=8
  dmf : Outport  Port=9
  wires:
  EngCylinder2/7 -> Sum2/2  "TqCyl2"
  EngCylinder7/7 -> Sum2/7  "TqCyl7"
  EngCylinder8/7 -> Sum2/8  "TqCyl8"
  EngCylinder6/7 -> Sum2/6  "TqCyl6"
  pTFScav/1 -> EngCylinder1/5(pTF_u), EngCylinder2/5, EngCylinder4/5, EngCylinder5/5, EngCylinder8/5, EngCylinder7/5, EngCylinder6/5, EngCylinder3/5
  EngCylinder3/7 -> Sum2/3  "TqCyl3"
  EngCylinder4/7 -> Sum2/4  "TqCyl4"
  EngCylinder5/7 -> Sum2/5  "TqCyl5"
  EngCylinder1/6(dmEmb_u) -> Sum1/1  "dmEmbInCyl1"
  EngCylinder2/5 -> Sum1/2  "dmEmbInCyl2"
  EngCylinder7/5 -> Sum1/7  "dmEmbInCyl7"
  EngCylinder3/5 -> Sum1/3  "dmEmbInCyl3"
  EngCylinder4/5 -> Sum1/4  "dmEmbInCyl4"
  EngCylinder6/5 -> Sum1/6  "dmEmbInCyl6"
  EngCylinder8/5 -> Sum1/8  "dmEmbInCyl8"
  EngCylinder5/5 -> Sum1/5  "dmEmbInCyl5"
  EngCylinder4/6 -> Sum/4  "dmEmbOutCyl4"
  EngCylinder3/6 -> Sum/3  "dmEmbOutCyl3"
  EngCylinder1/7(dmEmb_d) -> Sum/1  "dmEmbOutCyl1"
  EngCylinder7/6 -> Sum/7  "dmEmbOutCyl7"
  EngCylinder2/6 -> Sum/2  "dmEmbOutCyl2"
  EngCylinder6/6 -> Sum/6
  EngCylinder5/6 -> Sum/5  "dmEmbOutCyl5"
  EngCylinder8/4 -> Mux7/4  "dQCyl8"
  Mux7/1 -> Terminator7/1
  EngCylinder8/3 -> Mux7/3  "phiIg8"
  EngCylinder8/2 -> Mux7/2  "TCylWall8"
  EngCylinder8/1 -> Mux7/1  "phiCyl8"
  EngCylinder4/3 -> Mux3/3  "phiIg4"
  EngCylinder3/2 -> Mux2/2  "TCylWall3"
  Mux2/1 -> Terminator2/1
  EngCylinder5/2 -> Mux4/2  "TCylWall5"
  EngCylinder4/4 -> Mux3/4  "dQCyl4"
  EngCylinder4/1 -> Mux3/1  "phiCyl4"
  EngCylinder5/1 -> Mux4/1  "phiCyl5"
  Mux/1 -> Terminator/1
  Mux3/1 -> Terminator3/1
  EngCylinder3/1 -> Mux2/1  "phiCyl3"
  EngCylinder2/2 -> Mux1/2  "TCylWall2"
  EngCylinder2/3 -> Mux1/3  "phiIg2"
  EngCylinder4/2 -> Mux3/2  "TCylWall1"
  EngCylinder3/3 -> Mux2/3  "phiIg3"
  EngCylinder1/2(phi) -> pMaxFinder/1, Mux/1  "phiCyl1"
  EngCylinder3/4 -> Mux2/4  "dQCyl3"
  Mux4/1 -> Terminator4/1
  EngCylinder2/4 -> Mux1/4  "dQCyl2"
  EngCylinder5/4 -> Mux4/4  "dQCyl5"
  EngCylinder1/5(dQ) -> Mux/4  "dQCyl1"
  EngCylinder1/4(phiIg) -> Mux/3  "phiIg1"
  EngCylinder5/3 -> Mux4/3  "phiIg5"
  Mux1/1 -> Terminator1/1
  EngCylinder2/1 -> Mux1/1  "phiCyl2"
  EngCylinder1/3(teampWall) -> tempCyl1Wall/1, Mux/2  "TCylWall1"
  EngCylinder6/4 -> Mux5/4  "dQCyl6"
  Mux5/1 -> Terminator5/1
  EngCylinder6/3 -> Mux5/3  "phiIg6"
  pTFExh/1 -> EngCylinder1/6(pTF_d), EngCylinder8/6, EngCylinder7/6, EngCylinder6/6, EngCylinder5/6, EngCylinder4/6, EngCylinder3/6, EngCylinder2/6
  EngCylinder6/1 -> Mux5/1  "phiCyl6"
  EngCylinder6/2 -> Mux5/2  "TCylWall6"
  omega/1 -> EngCylinder1/7(omega), EngCylinder3/7, EngCylinder4/7, EngCylinder5/7, EngCylinder6/7, EngCylinder7/7, EngCylinder8/7, EngCylinder2/7
  EngCylinder7/1 -> Mux6/1  "phiCyl7"
  EngCylinder1/8(Tq) -> Sum2/1  "TqCyl1"
  EngCylinder7/4 -> Mux6/4  "dQCyl7"
  EngCylinder7/2 -> Mux6/2  "TCylWall7"
  EngCylinder8/6 -> Sum/8  "dmEmbOutCyl8"
  EngCylinder7/3 -> Mux6/3  "phiIg7"
  Mux6/1 -> Terminator6/1
  Sum2/1 -> Tq/1
  Sum1/1 -> dmEmbScvg/1
  Sum/1 -> dmEmbExh/1
  pMaxFinder/1 -> pMax/1  "pMax"
  pMaxFinder/2 -> Terminator8/1
  EngCylinder1/1(pCyl) -> pCyl/1, pMaxFinder/2  "phiCyl1"
  EngCylinder1/9(exhVVAOpen) -> exhVVAOpenCyl/1
  EngCylinder1/10(vCyl) -> vCyl/1
  EngCylinder1/11(dmb) -> Sum3/1  "dmf1"
  EngCylinder2/8 -> Sum3/2  "dmf2"
  EngCylinder3/8 -> Sum3/3  "dmf3"
  EngCylinder4/8 -> Sum3/4  "dmf4"
  EngCylinder5/8 -> Sum3/5  "dmf5"
  EngCylinder6/8 -> Sum3/6  "dmf6"
  EngCylinder7/8 -> Sum3/7  "dmf7"
  EngCylinder8/8 -> Sum3/8  "dmf8"
  Sum3/1 -> dmf/1  "dmfTot"
  uGov/1 -> Mux8/1
  phiInj/1 -> Mux8/2
  cAStartNom/1 -> Mux8/3
  dCALiftUp/1 -> Mux8/4
  Mux8/1 -> [ctrlSig]
  [ctrlSig] -> Demux/1
  Demux/1 -> EngCylinder1/1(uGov)
  Demux/2 -> EngCylinder1/2(phiInj)
  Demux/3 -> EngCylinder1/3(cAStartNom)
  Demux/4 -> EngCylinder1/4(dCALiftUp)
  [ctrlSig] -> Demux1/1
  Demux1/1 -> EngCylinder2/1
  Demux1/2 -> EngCylinder2/2
  Demux1/3 -> EngCylinder2/3
  Demux1/4 -> EngCylinder2/4
  [ctrlSig] -> Demux2/1
  Demux2/1 -> EngCylinder3/1
  Demux2/2 -> EngCylinder3/2
  Demux2/3 -> EngCylinder3/3
  Demux2/4 -> EngCylinder3/4
  [ctrlSig] -> Demux3/1
  Demux3/1 -> EngCylinder4/1
  Demux3/2 -> EngCylinder4/2
  Demux3/3 -> EngCylinder4/3
  Demux3/4 -> EngCylinder4/4
  [ctrlSig] -> Demux4/1
  Demux4/1 -> EngCylinder5/1
  Demux4/2 -> EngCylinder5/2
  Demux4/3 -> EngCylinder5/3
  Demux4/4 -> EngCylinder5/4
  [ctrlSig] -> Demux5/1
  Demux5/1 -> EngCylinder6/1
  Demux5/2 -> EngCylinder6/2
  Demux5/3 -> EngCylinder6/3
  Demux5/4 -> EngCylinder6/4
  [ctrlSig] -> Demux6/1
  Demux6/1 -> EngCylinder7/1
  Demux6/2 -> EngCylinder7/2
  Demux6/3 -> EngCylinder7/3
  Demux6/4 -> EngCylinder7/4
  [ctrlSig] -> Demux7/1
  Demux7/1 -> EngCylinder8/1
  Demux7/2 -> EngCylinder8/2
  Demux7/3 -> EngCylinder8/3
  Demux7/4 -> EngCylinder8/4

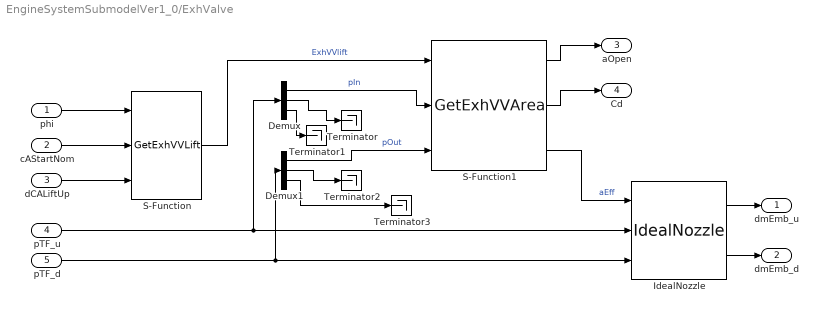
== system EngineSystemSubmodelVer1_0/ExhValve ==
  phi : Inport
  cAStartNom : Inport  Port=2
  dCALiftUp : Inport  Port=3
  pTF_u : Inport  Port=4
  pTF_d : Inport  Port=5
  Demux : Demux  Outputs=3
  Demux1 : Demux  Outputs=3
  IdealNozzle : EngineSystemSubmodel/IdealNozzle  fs=fs
  S-Function : S-Function  FunctionName=GetExhVVLift  Parameters=liftMax,cAStartRef,dCALiftUp,dCALiftDown,dCALiftTopRef,cAVVUpRef,cAVVDownRef,liftUpRef,liftDownRef  EnableBusSupport=off  mask{liftMax=liftMax, cAStartRef=cAStartRef, dCALiftUp=dCALiftUp, dCALiftDown=dCALiftDown, dCALiftTopRef=dCALiftTopRef, cAVVUpRef=cAVVUpRef, cAVVDownRef=cAVVDownRef, liftUpRef=liftUpRef, liftDownRef=liftDownRef}
      mask prompts: liftMax "Maximum valve lift [m]"; cAStartRef "Crank angle at the beginning of valve lift [deg]"; dCALiftUp "Duration for valve lifting [deg]"; dCALiftDown "Duration for valve closing [deg]"; dCALiftTopRef "Duration for valve fully opened [deg]"; cAVVUpRef "Crank angle array reference for valve opening [deg]"; cAVVDownRef "Crank angle array reference for valve closing [deg]"; liftUpRef "Normalized lift reference for valve opening (0~1)"; liftDownRef "Normalized lift reference for valve closing (0~1)"
  S-Function1 : S-Function  FunctionName=GetExhVVArea  Parameters=Dv,beta,w,Dp,Ds,coeffCdCorrP,coeffCdCorrQ,coeffCdCorrPR  EnableBusSupport=off  mask{Dv=Dv, beta=beta, w=w, Dp=Dp, Ds=Ds, coeffCdCorrP=[0.5329;-0.2047;0.04292], coeffCdCorrQ=[0.5359;-0.2962;0.06275], coeffCdCorrPR=[-0.006345;0.09503;0.8117]}
      mask prompts: Dv "Valve head diameter"; beta "Seat angle"; w "Valve seat width"; Dp "Inner seat diameter"; Ds "Stem diameter"; coeffCdCorrP "Produt coefficient for discharge coefficient for lift ratio"; coeffCdCorrQ "Quotient coefficient for discharge coefficient for lift ratio"; coeffCdCorrPR "Coefficient for discharge coefficient for pressure ratio"
  Terminator{,1..3} (4 alike) : Terminator
  dmEmb_u : Outport
  dmEmb_d : Outport  Port=2
  aOpen : Outport  Port=3
  Cd : Outport  Port=4
  wires:
  S-Function/1 -> S-Function1/1  "ExhVVlift"
  pTF_d/1 -> Demux1/1, IdealNozzle/3
  pTF_u/1 -> Demux/1, IdealNozzle/2
  IdealNozzle/2 -> dmEmb_d/1
  IdealNozzle/1 -> dmEmb_u/1
  phi/1 -> S-Function/1
  cAStartNom/1 -> S-Function/2
  dCALiftUp/1 -> S-Function/3
  S-Function1/3 -> IdealNozzle/1  "aEff"
  S-Function1/1 -> aOpen/1
  S-Function1/2 -> Cd/1
  Demux/1 -> S-Function1/2  "pIn"
  Demux1/1 -> S-Function1/3  "pOut"
  Demux/2 -> Terminator/1
  Demux/3 -> Terminator1/1
  Demux1/2 -> Terminator2/1
  Demux1/3 -> Terminator3/1

== system EngineSystemSubmodelVer1_0/Governor ==
  u saturated : Inport
  omega_pu : Inport  Port=2
  "wNL, pu" : Inport  Port=3
  "pe, pu" : Inport  Port=4
  Constant : Constant
  Gain : Gain  Gain=genset.governor.droop
  PID controller : Subsystem
  Product : Product  RndMeth=Zero
  Sum : Sum  Inputs=|+-
  Sum1 : Sum  Inputs=|+-
  u : Outport
  wires:
  omega_pu/1 -> PID controller/2(omega_pu), Sum/2
  "pe, pu"/1 -> Gain/1
  u saturated/1 -> PID controller/3(u saturated)
  Sum1/1 -> Product/2
  Constant/1 -> Sum1/1
  "wNL, pu"/1 -> Product/1
  Product/1 -> Sum/1
  Sum/1 -> PID controller/1(e)
  Gain/1 -> Sum1/2
  PID controller/1(u) -> u/1  "u"

== system EngineSystemSubmodelVer1_0/Governor_SpeedControl ==
  u saturated : Inport
  omega_pu : Inport  Port=2
  omega_pu_ref : Inport  Port=3
  PID controller : Subsystem  mask{Kp=Kp, Kd=Kd, N=N, Ki=Ki, Kb=Kb, omega0=omega0, u_max=u_max, u_min=u_min, u0=u0}
      mask prompts: Kp "Proportional gain"; Kd "Differtial gain"; N "Dirty derivative gain"; Ki "Integral gain"; Kb "Back-calculation gain"; omega0 "Initial speed"; u_max "Maximum output"; u_min "Minimum output"; u0 "Initial output"
  Sum : Sum  Inputs=|+-
  u : Outport
  wires:
  omega_pu/1 -> PID controller/2(omega_pu), Sum/2
  u saturated/1 -> PID controller/3(u saturated)
  omega_pu_ref/1 -> Sum/1
  Sum/1 -> PID controller/1(e)  "error"
  PID controller/1(u) -> u/1

== system EngineSystemSubmodelVer1_0/IdealNozzle ==
  A_eff : Inport
  pTF_u : Inport  Port=2
  pTF_d : Inport  Port=3
  Bus Creator : BusCreator  Inputs=3
  Bus Creator1 : BusCreator  Inputs=3
  Bus Selector : BusSelector  OutputSignals=p,T,F
  Bus Selector1 : BusSelector  OutputSignals=p,T,F
  S-Function : S-Function  FunctionName=IdealNozzlePTF  Parameters=fs  SFunctionModules='GetIdealNozzleFlw GetThdynCombGasZach GetCompCombGas_rtutil'  EnableBusSupport=off
  dmEmb_u : Outport
  dmEmb_d : Outport  Port=2
  wires:
  Bus Creator1/1 -> dmEmb_d/1
  S-Function/6 -> Bus Creator1/3  "dmbd"
  S-Function/5 -> Bus Creator1/2  "dEd"
  S-Function/4 -> Bus Creator1/1  "dmd"
  Bus Creator/1 -> dmEmb_u/1
  S-Function/3 -> Bus Creator/3  "dmbu"
  S-Function/2 -> Bus Creator/2  "dEu"
  S-Function/1 -> Bus Creator/1  "dmu"
  Bus Selector1/1 -> S-Function/5  "<p>"
  Bus Selector1/3 -> S-Function/7  "<F>"
  Bus Selector1/2 -> S-Function/6  "<T>"
  Bus Selector/1 -> S-Function/2  "<p>"
  Bus Selector/2 -> S-Function/3  "<T>"
  Bus Selector/3 -> S-Function/4  "<F>"
  A_eff/1 -> S-Function/1
  pTF_u/1 -> Bus Selector/1
  pTF_d/1 -> Bus Selector1/1

== system EngineSystemSubmodelVer1_0/InCylinderMV ==
  PTFu : Inport
  PTFd : Inport  Port=2
  omegae : Inport  Port=3
  throttle : Inport  Port=4
  Demux : Demux  Outputs=3
  Demux1 : Demux  Outputs=3
  Mux : Mux  Inputs=3
  Mux1 : Mux  Inputs=3
  S-Function : S-Function  FunctionName=InCylinderMV  Parameters=fs,Vd,LHV,Pe_nom,SFC,vol_eff_coeff1,vol_eff_coeff2,T_pe,nstroke,m_f_cyc_max,C1,p_a_inf,Pe0  SFunctionModules='GetThdynCombGasZach'  EnableBusSupport=off  mask{fs=fs, Vd=Vd, LHV=LHV, Pe_nom=Pe_nom, SFC=SFC, vol_eff_coeff1=vol_eff_coeff1, vol_eff_coeff2=vol_eff_coeff2, T_pe=T_pe, nstroke=nstroke, m_f_cyc_max=m_f_cyc_max, C1=C1, p_a_inf=p_a_inf, Pe0=Pe0}
      mask prompts: fs "Stoichiometric fuel air ratio"; Vd "Displacement volume [m3]"; LHV "Low heating value of the fuel [J/kg]"; Pe_nom "Rated power [W]"; SFC "Coefficient for the SFC model"; vol_eff_coeff1 "Coefficient for volumetric efficiency model for higher pressure"; vol_eff_coeff2 "Coefficient for volumetric efficiency model for lower pressure"; T_pe "Time constant for power development (0.01)"; nstroke "Number of stroke"; m_f_cyc_max "Maximum injected fuel per cycle"; C1 "Cofficient of heat transfer"; p_a_inf "Upper pressure limit for vol. eff. model change"; Pe0 "Initial power load"
  dmEmbu : Outport
  dmEmbd : Outport  Port=2
  Tqe : Outport  Port=3
  vol_eff : Outport  Port=4
  pe_pu : Outport  Port=5
  wires:
  S-Function/8 -> vol_eff/1
  S-Function/7 -> Tqe/1
  Mux1/1 -> dmEmbd/1
  S-Function/6 -> Mux1/3
  S-Function/5 -> Mux1/2
  S-Function/4 -> Mux1/1
  Mux/1 -> dmEmbu/1
  S-Function/3 -> Mux/3
  S-Function/2 -> Mux/2
  S-Function/1 -> Mux/1
  throttle/1 -> S-Function/8
  omegae/1 -> S-Function/7
  Demux1/3 -> S-Function/6
  Demux1/2 -> S-Function/5
  Demux1/1 -> S-Function/4
  PTFd/1 -> Demux1/1
  Demux/3 -> S-Function/3
  Demux/2 -> S-Function/2
  Demux/1 -> S-Function/1
  PTFu/1 -> Demux/1
  S-Function/9 -> pe_pu/1

== system EngineSystemSubmodelVer1_0/InCylinderMV1 ==
  pTFu : Inport
  pTFd : Inport  Port=2
  omegae : Inport  Port=3
  throttle : Inport  Port=4
  Bus Creator : BusCreator  Inputs=3
  Bus Creator1 : BusCreator  Inputs=3
  Bus Selector : BusSelector  OutputSignals=p,T,F
  Bus Selector1 : BusSelector  OutputSignals=p,T,F
  S-Function : S-Function  FunctionName=InCylinderMV  Parameters=fs,Vd,LHV,Pe_nom,SFC,vol_eff_coeff1,vol_eff_coeff2,T_pe,nstroke,m_f_cyc_max,C1,p_a_inf,Pe0  SFunctionModules='GetThdynCombGasZach'  EnableBusSupport=off  mask{fs=fs, Vd=Vd, LHV=LHV, Pe_nom=Pe_nom, SFC=SFC, vol_eff_coeff1=vol_eff_coeff1, vol_eff_coeff2=vol_eff_coeff2, T_pe=T_pe, nstroke=nstroke, m_f_cyc_max=m_f_cyc_max, C1=C1, p_a_inf=p_a_inf, Pe0=Pe0}
      mask prompts: fs "Stoichiometric fuel air ratio"; Vd "Displacement volume [m3]"; LHV "Low heating value of the fuel [J/kg]"; Pe_nom "Rated power [W]"; SFC "Coefficient for the SFC model"; vol_eff_coeff1 "Coefficient for volumetric efficiency model for higher pressure"; vol_eff_coeff2 "Coefficient for volumetric efficiency model for lower pressure"; T_pe "Time constant for power development (0.01)"; nstroke "Number of stroke"; m_f_cyc_max "Maximum injected fuel per cycle"; C1 "Cofficient of heat transfer"; p_a_inf "Upper pressure limit for vol. eff. model change"; Pe0 "Initial power load"
  dmEmbu : Outport
  dmEmbd : Outport  Port=2
  Tqe : Outport  Port=3
  vol_eff : Outport  Port=4
  pe_pu : Outport  Port=5
  wires:
  S-Function/8 -> vol_eff/1  "volEff"
  S-Function/7 -> Tqe/1
  Bus Creator1/1 -> dmEmbd/1
  Bus Creator/1 -> dmEmbu/1
  S-Function/3 -> Bus Creator/3  "dmbu"
  S-Function/2 -> Bus Creator/2  "dEu"
  S-Function/1 -> Bus Creator/1  "dmu"
  throttle/1 -> S-Function/8
  omegae/1 -> S-Function/7
  S-Function/9 -> pe_pu/1
  S-Function/4 -> Bus Creator1/1  "dmd"
  S-Function/6 -> Bus Creator1/3  "dmbd"
  S-Function/5 -> Bus Creator1/2  "dEd"
  pTFu/1 -> Bus Selector/1
  pTFd/1 -> Bus Selector1/1
  Bus Selector/2 -> S-Function/2  "<T>"
  Bus Selector/1 -> S-Function/1  "<p>"
  Bus Selector/3 -> S-Function/3  "<F>"
  Bus Selector1/2 -> S-Function/5  "<T>"
  Bus Selector1/1 -> S-Function/4  "<p>"
  Bus Selector1/3 -> S-Function/6  "<F>"

== system EngineSystemSubmodelVer1_0/IntakePort ==
  phi : Inport
  pTF_u : Inport  Port=2
  pTF_d : Inport  Port=3
  IdealNozzle : EngineSystemSubmodel/IdealNozzle  fs=fs
  S-Function : S-Function  FunctionName=GetInportArea  Parameters=nStroke,aCrank,lambdaCrank,X,Y,r,nPort,stroke  EnableBusSupport=off  mask{nStroke=nStroke, aCrank=aCrank, lambdaCrank=lambdaCrank, X=X, Y=Y, r=r, nPort=nPort, stroke=stroke}
      mask prompts: nStroke "Number of stroke"; aCrank "Length of crank rod (stroke /2) [m]"; lambdaCrank "Ratio of length of a crank rod to a connecting rod"; X "Width of a port [m]"; Y "Height of a port [m]"; r "Radius of a fillet of a port [m]"; nPort "Number of port [pcs]"; stroke "Length of stroke [m]"
  dmEmb_u : Outport
  dmEmb_d : Outport  Port=2
  aOpen : Outport  Port=3
  Cd : Outport  Port=4
  xP : Outport  Port=5
  wires:
  S-Function/2 -> Cd/1
  S-Function/1 -> aOpen/1
  pTF_d/1 -> IdealNozzle/3
  pTF_u/1 -> IdealNozzle/2
  IdealNozzle/2 -> dmEmb_d/1
  IdealNozzle/1 -> dmEmb_u/1
  phi/1 -> S-Function/1
  S-Function/3 -> IdealNozzle/1  "aEff"
  S-Function/4 -> xP/1

== system EngineSystemSubmodelVer1_0/Load ==
  input : Inport
  Constant : Constant  Value=Load_bias
  Constant2 : Constant  Value=Load_index
  From Workspace : FromWorkspace  VariableName=Tq_hist  SampleTime=0
  Multiport Switch : MultiPortSwitch  Inputs=6
  Ramp : simulink/Sources/Ramp  slope=Load_amp  start=Start_time  X0=Load_bias
  Sine Wave : Sin  Amplitude=Load_amp  Bias=Load_bias  Frequency=2*pi/T_load  SampleTime=0
  Step : Step  Time=Start_time  Before=Load_bias  After=Load_amp  SampleTime=0
  Transport Delay : TransportDelay  DelayTime=Start_time  InitialOutput=Load_bias
  Transport Delay1 : TransportDelay  DelayTime=Start_time  InitialOutput=Load_bias
  Transport Delay2 : TransportDelay  DelayTime=Start_time  InitialOutput=Load_bias
  Out1 : Outport
  wires:
  Constant2/1 -> Multiport Switch/1
  input/1 -> Transport Delay2/1
  Transport Delay/1 -> Multiport Switch/3
  Transport Delay2/1 -> Multiport Switch/6
  Transport Delay1/1 -> Multiport Switch/5
  Step/1 -> Multiport Switch/2
  Sine Wave/1 -> Transport Delay/1
  Multiport Switch/1 -> Out1/1
  Constant/1 -> Multiport Switch/7
  Ramp/1 -> Multiport Switch/4
  From Workspace/1 -> Transport Delay1/1
